simulink model "ModelMatematyczny"  (R2015a)
settings: Solver=ode45  StartTime=0.0  StopTime=10.0  RelTol=1e-3
values from neighbouring files (symbols this model uses):
  a = 31    [stale.m]
  b = 40    [stale.m]
  c = 10    [stale.m]
  H2max = 40    [stale.m]
  R = 40    [stale.m]
  w = 5    [stale.m]
undefined symbols (not defined in the file or in its folder): C1, C2, C3, q
settings Model: Creator=Student  LastModifiedBy=Student

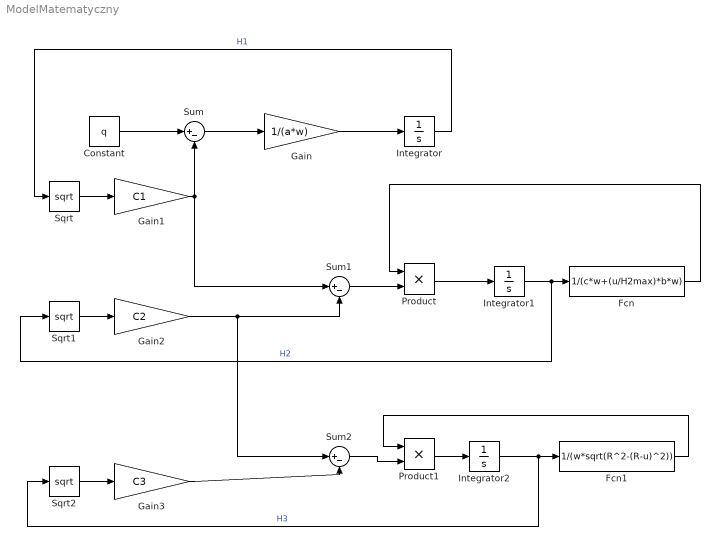
== system ModelMatematyczny ==
  Constant : Constant  Value=q
  Fcn : Fcn  Expr=1/(c*w+(u/H2max)*b*w)
  Fcn1 : Fcn  Expr=1/(w*sqrt(R^2-(R-u)^2))
  Gain : Gain  Gain=1/(a*w)
  Gain1 : Gain  Gain=C1
  Gain2 : Gain  Gain=C2
  Gain3 : Gain  Gain=C3
  Integrator : Integrator
  Integrator1 : Integrator
  Integrator2 : Integrator
  Product : Product
  Product1 : Product
  Sqrt : Sqrt  SaturateOnIntegerOverflow=on
  Sqrt1 : Sqrt  SaturateOnIntegerOverflow=on
  Sqrt2 : Sqrt  SaturateOnIntegerOverflow=on
  Sum : Sum  Inputs=|+-
  Sum1 : Sum  Inputs=|+-
  Sum2 : Sum  Inputs=|+-
  wires:
  Sum/1 -> Gain/1
  Constant/1 -> Sum/1
  Sqrt/1 -> Gain1/1
  Gain1/1 -> Sum/2, Sum1/1
  Integrator/1 -> Sqrt/1  "H1"
  Gain/1 -> Integrator/1
  Integrator1/1 -> Sqrt1/1, Fcn/1  "H2"
  Fcn/1 -> Product/1
  Sqrt1/1 -> Gain2/1
  Gain2/1 -> Sum2/1, Sum1/2
  Sum1/1 -> Product/2
  Product/1 -> Integrator1/1
  Integrator2/1 -> Sqrt2/1, Fcn1/1  "H3"
  Sqrt2/1 -> Gain3/1
  Gain3/1 -> Sum2/2
  Sum2/1 -> Product1/2
  Product1/1 -> Integrator2/1
  Fcn1/1 -> Product1/1
